simulink model "PostLab"  (R2025b)
settings: Solver=VariableStepAuto  StartTime=0.0  StopTime=120  RelTol=1e-3
InitFcn:
  | m = 5;
  | g = 9.81;
  | mu = 0;
  | K = 1000;
  | A = 5e-4;
  | R1 = 10^10;
  | R2 = R1;
  | p1 = 2*10^5;
  | p2 = p1;
  | rou = 1;
settings Model: Creator=Murl0  LastModifiedBy=Murl0

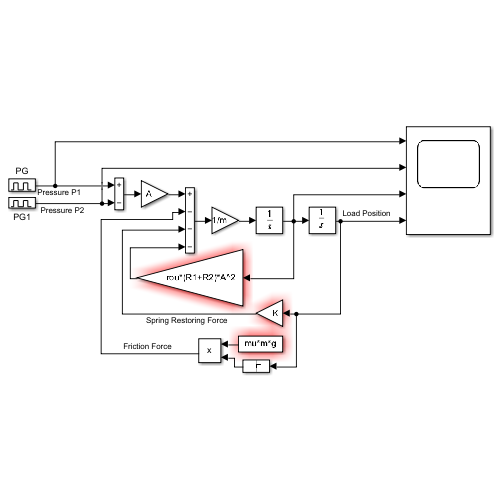
[thumbnail: Simulink's stored preview of the top-level diagram]
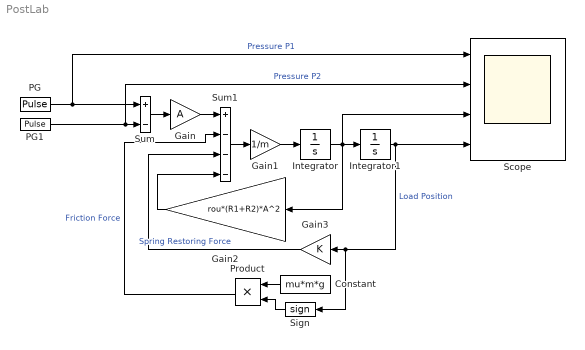
== system PostLab ==
  Constant : Constant  Value=mu*m*g
  Gain : Gain  Gain=A
  Gain1 : Gain  Gain=1/m
  Gain2 : Gain  Gain=rou*(R1+R2)*A^2
  Gain3 : Gain  Gain=K
  Integrator : Integrator
  Integrator1 : Integrator
  PG : DiscretePulseGenerator  PulseType=Time based  Amplitude=p1  Period=60  PulseWidth=50
  PG1 : DiscretePulseGenerator  PulseType=Time based  Amplitude=p2  Period=60  PulseWidth=50  PhaseDelay=30
  Product : Product
  Scope : Scope  NumInputPorts=4
      settings: ActiveDisplayYMinimum=-24999.999999999993  ActiveDisplayYMaximum=225000
  Sign : Signum
  Sum : Sum  Inputs=+-
  Sum1 : Sum  Inputs=+---
  wires:
  PG/1 -> Sum/1, Scope/1  "Pressure P1"
  PG1/1 -> Scope/2, Sum/2  "Pressure P2"
  Sum/1 -> Gain/1
  Gain/1 -> Sum1/1
  Sum1/1 -> Gain1/1
  Gain1/1 -> Integrator/1
  Integrator/1 -> Scope/3, Gain2/1, Integrator1/1
  Gain2/1 -> Sum1/4
  Integrator1/1 -> Sign/1, Gain3/1, Scope/4  "Load Position"
  Gain3/1 -> Sum1/3  "Spring Restoring Force"
  Constant/1 -> Product/1
  Sign/1 -> Product/2
  Product/1 -> Sum1/2  "Friction Force"
